simulink library "fsr"  (Simulink 8.1)
settings: Solver=ode45  StartTime=0.0  StopTime=10.0  RelTol=1e-3
undefined symbols (not defined in the file or in its folder): FALSE, KJUD_FCWMaxActSpeed_kph, KJUD_FCWMaxDeactSpeed_kph, KJUD_FCWMinActSpeed_kph, KJUD_FCWMinDeactSpeed_kph, TRUE
settings Model: Creator=xsellart  LastModifiedBy=tescamilla

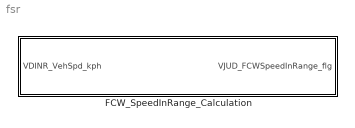
== system fsr ==
  FCW_SpeedInRange_Calculation : Subsystem

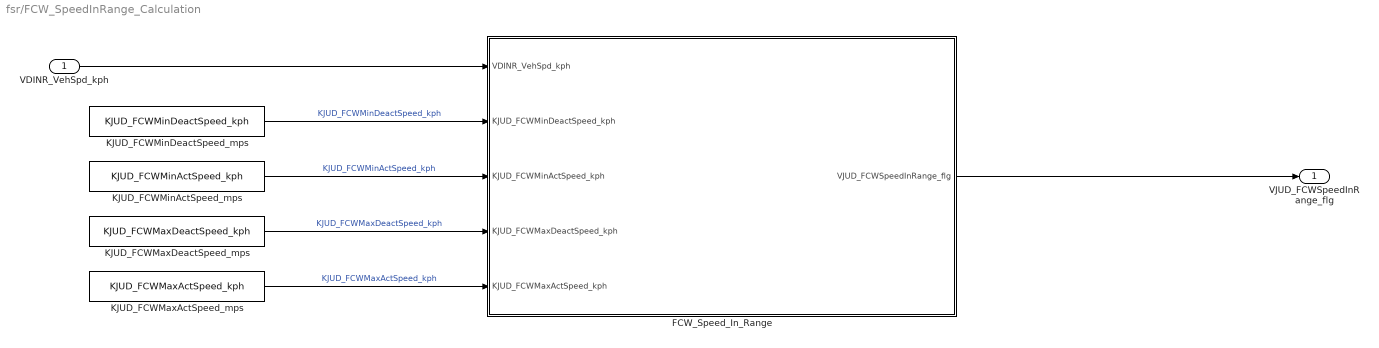
== system fsr/FCW_SpeedInRange_Calculation ==
  VDINR_VehSpd_kph : Inport
  FCW_Speed_In_Range : Stateflow chart  TreatAsAtomicUnit=on
  KJUD_FCWMaxActSpeed_mps : Constant  Value=KJUD_FCWMaxActSpeed_kph
  KJUD_FCWMaxDeactSpeed_mps : Constant  Value=KJUD_FCWMaxDeactSpeed_kph
  KJUD_FCWMinActSpeed_mps : Constant  Value=KJUD_FCWMinActSpeed_kph
  KJUD_FCWMinDeactSpeed_mps : Constant  Value=KJUD_FCWMinDeactSpeed_kph
  VJUD_FCWSpeedInRange_flg : Outport
  wires:
  VDINR_VehSpd_kph/1 -> FCW_Speed_In_Range/1(VDINR_VehSpd_kph)
  FCW_Speed_In_Range/1(VJUD_FCWSpeedInRange_flg) -> VJUD_FCWSpeedInRange_flg/1
  KJUD_FCWMinDeactSpeed_mps/1 -> FCW_Speed_In_Range/2(KJUD_FCWMinDeactSpeed_kph)  "KJUD_FCWMinDeactSpeed_kph"
  KJUD_FCWMinActSpeed_mps/1 -> FCW_Speed_In_Range/3(KJUD_FCWMinActSpeed_kph)  "KJUD_FCWMinActSpeed_kph"
  KJUD_FCWMaxActSpeed_mps/1 -> FCW_Speed_In_Range/5(KJUD_FCWMaxActSpeed_kph)  "KJUD_FCWMaxActSpeed_kph"
  KJUD_FCWMaxDeactSpeed_mps/1 -> FCW_Speed_In_Range/4(KJUD_FCWMaxDeactSpeed_kph)  "KJUD_FCWMaxDeactSpeed_kph"

== stateflow chart FCW_SpeedInRange_Calculation/FCW_Speed_In_Range ==
  state SPEED_OUT_RANGE
    en:
    VJUD_FCWSpeedInRange_flg = FALSE;
  state SPEED_IN_RANGE
    en:
    VJUD_FCWSpeedInRange_flg = TRUE;
  (default) -> SPEED_OUT_RANGE
  SPEED_OUT_RANGE -> SPEED_IN_RANGE : [(VDINR_VehSpd_kph>KJUD_FCWMinActSpeed_kph) &&...
      | (VDINR_VehSpd_kph<KJUD_FCWMaxActSpeed_kph)]
  SPEED_IN_RANGE -> SPEED_OUT_RANGE : [(VDINR_VehSpd_kph>KJUD_FCWMaxDeactSpeed_kph) ||...
      | (VDINR_VehSpd_kph<KJUD_FCWMinDeactSpeed_kph)]
  data: VDINR_VehSpd_kph input single; KJUD_FCWMinDeactSpeed_kph input single; VJUD_FCWSpeedInRange_flg output boolean; KJUD_FCWMinActSpeed_kph input single; KJUD_FCWMaxDeactSpeed_kph input single; KJUD_FCWMaxActSpeed_kph input single; TRUE parameter boolean; FALSE parameter boolean
